simulink model "model"  (R2021a)
settings: Solver=VariableStepAuto  StartTime=0.0  StopTime=10.0  RelTol=1e-3
values from neighbouring files (symbols this model uses):
  namp = n    [script_main.m]    (also in skryptv1.m = 0.005; skryptv2.m)
  non = 1    [script_main.m]    (also in skryptv1.m = 0; skryptv2.m)
  Ts = 1e-2    (= 0.01)    [script_main.m]    (also in skryptv1.m; skryptv2.m)
libraries: cstblocks x1
settings Model: Creator=mokro  LastModifiedBy=mokro

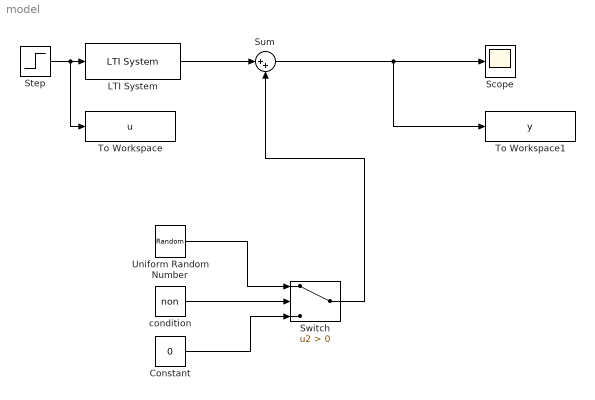
== system model ==
  Constant : Constant  Value=0
  LTI System : cstblocks/LTI System  sys=G  IC=[]
  Scope : Scope
  Step : Step  SampleTime=0
  Sum : Sum  Inputs=|++
  Switch : Switch  Criteria=u2 > Threshold
  To Workspace : ToWorkspace  VariableName=u  SaveFormat=Timeseries  SampleTime=Ts
  To Workspace1 : ToWorkspace  VariableName=y  SaveFormat=Timeseries  SampleTime=Ts
  Uniform Random Number : UniformRandomNumber  Minimum=-namp  Maximum=namp  SampleTime=Ts
  condition : Constant  Value=non
  wires:
  Step/1 -> To Workspace/1, LTI System/1
  Sum/1 -> To Workspace1/1, Scope/1
  LTI System/1 -> Sum/1
  Uniform Random Number/1 -> Switch/1
  Switch/1 -> Sum/2
  Constant/1 -> Switch/3
  condition/1 -> Switch/2
